simulink subsystem "XinSVSF3rd"  (R2020b)
settings: Solver=VariableStepAuto  StartTime=0.0  StopTime=10.0  RelTol=1e-3
values from neighbouring files (symbols this model uses):
  DeltaT = 0.1    [IMM_SVSF_VBL_init.m]
  Eta = 1    [IMM_SVSF_VBL_init.m]
  Gamma = .38    (= 0.38)    [IMM_SVSF_VBL_init.m]
  Psi = 3.2    [IMM_SVSF_VBL_init.m]
  Q = diag([1e-8,1e-8,1e-8,1e-10,1e-10,1e-10])    [IMM_SVSF_VBL_init.m]
  R = [.5e-2 0;0  9.5e-2]    [IMM_SVSF_VBL_init.m]
undefined symbols (not defined in the file or in its folder): A
libraries: dspmtrx3 x4, dspinverses x1
settings Model: Creator=Sara  LastModifiedBy=Sara

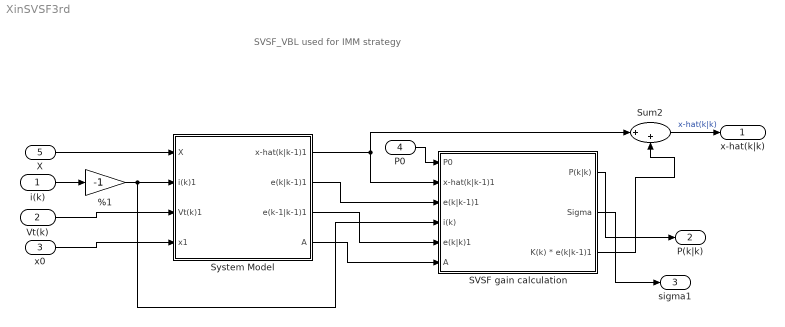
== system XinSVSF3rd ==
  note: SVSF_VBL used for IMM strategy
  i(k) : Inport
  Vt(k) : Inport  Port=2
  x0 : Inport  Port=3
  P0 : Inport  Port=4
  X : Inport  Port=5
  %1 : Gain  Gain=-1  SampleTime=DeltaT
  SVSF gain calculation : Subsystem
  Sum2 : Sum  Inputs=|++  SampleTime=DeltaT
  System Model : Subsystem
  x-hat(k|k) : Outport  VectorParamsAs1DForOutWhenUnconnected=off
  P(k|k) : Outport  Port=2
  sigma1 : Outport  Port=3
  wires:
  System Model/2(e(k|k-1)1) -> SVSF gain calculation/3(e(k|k-1)1)
  P0/1 -> SVSF gain calculation/1(P0)
  System Model/1(x-hat(k|k-1)1) -> SVSF gain calculation/2(x-hat(k|k-1)1), Sum2/1
  SVSF gain calculation/2(Sigma) -> sigma1/1
  System Model/3(e(k-1|k-1)1) -> SVSF gain calculation/5(e(k|k)1)
  SVSF gain calculation/3(K(k) * e(k|k-1)1) -> Sum2/2
  Sum2/1 -> x-hat(k|k)/1  "x-hat(k|k)"
  Vt(k)/1 -> System Model/3(Vt(k)1)
  SVSF gain calculation/1(P(k|k)) -> P(k|k)/1
  %1/1 -> System Model/2(i(k)1), SVSF gain calculation/4(i(k))
  x0/1 -> System Model/4(x1)
  System Model/4(A) -> SVSF gain calculation/6(A)
  X/1 -> System Model/1(X)
  i(k)/1 -> %1/1

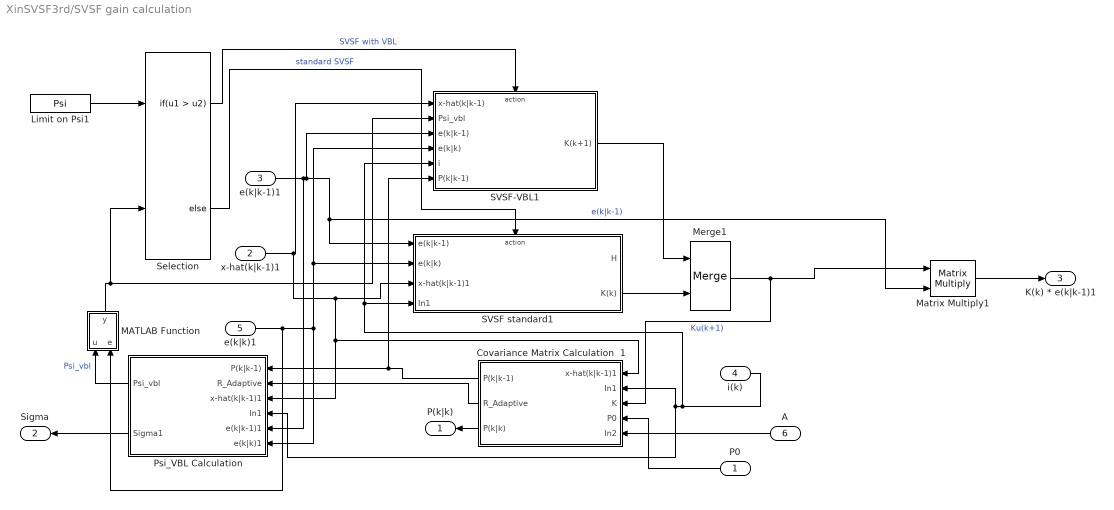
== system XinSVSF3rd/SVSF gain calculation ==
  P0 : Inport
  x-hat(k|k-1)1 : Inport  Port=2
  e(k|k-1)1 : Inport  Port=3
  i(k) : Inport  Port=4
  e(k|k)1 : Inport  Port=5
  A : Inport  Port=6
  " SVSF-VBL1" : Subsystem  TreatAsAtomicUnit=on
  " Selection" : If  NumInputs=2  IfExpression=u1 > u2
  Covariance Matrix Calculation  1 : Subsystem
  Limit on Psi1 : Constant  Value=Psi  SampleTime=DeltaT
  MATLAB Function : MATLAB Function  TreatAsAtomicUnit=on
  Matrix Multiply1 : Product  Multiplication=Matrix(*)
  Merge1 : Merge
  Psi_VBL Calculation : Subsystem
  SVSF standard1 : Subsystem
  P(k|k) : Outport
  Sigma : Outport  Port=2
  K(k) * e(k|k-1)1 : Outport  Port=3
  wires:
  Psi_VBL Calculation/2(Sigma1) -> Sigma/1
  Covariance Matrix Calculation  1/3("P(k|k) ") -> P(k|k)/1
  P0/1 -> Covariance Matrix Calculation  1/4(P0)
  e(k|k-1)1/1 -> SVSF standard1/1(e(k|k-1)), Matrix Multiply1/2, " SVSF-VBL1"/3(e(k|k-1)), Psi_VBL Calculation/5(e(k|k-1)1)  "e(k|k-1)"
  Psi_VBL Calculation/1(Psi_vbl) -> MATLAB Function/1(u)  "Psi_vbl"
  Covariance Matrix Calculation  1/1(P(k|k-1)) -> " SVSF-VBL1"/6(P(k|k-1)), Psi_VBL Calculation/1(P(k|k-1))
  SVSF standard1/2(K(k)) -> Merge1/2
  Limit on Psi1/1 -> " Selection"/1
  e(k|k)1/1 -> SVSF standard1/2(e(k|k)), " SVSF-VBL1"/4(e(k|k)), Psi_VBL Calculation/6(e(k|k)1), MATLAB Function/2(e)
  " Selection"/2 -> SVSF standard1/Action  "standard SVSF"
  Merge1/1 -> Matrix Multiply1/1, Covariance Matrix Calculation  1/3(K)  "Ku(k+1)"
  " SVSF-VBL1"/1(K(k+1)) -> Merge1/1
  x-hat(k|k-1)1/1 -> SVSF standard1/3(x-hat(k|k-1)1), Covariance Matrix Calculation  1/1(x-hat(k|k-1)1), Psi_VBL Calculation/3(x-hat(k|k-1)1), " SVSF-VBL1"/1(x-hat(k|k-1))
  i(k)/1 -> Covariance Matrix Calculation  1/2(In1), Psi_VBL Calculation/4(In1), SVSF standard1/4(In1), " SVSF-VBL1"/5(i)
  Matrix Multiply1/1 -> K(k) * e(k|k-1)1/1
  " Selection"/1 -> " SVSF-VBL1"/Action  "SVSF with VBL"
  Covariance Matrix Calculation  1/2(R_Adaptive) -> Psi_VBL Calculation/2(R_Adaptive)
  MATLAB Function/1(y) -> " Selection"/2, " SVSF-VBL1"/2(Psi_vbl)
  A/1 -> Covariance Matrix Calculation  1/5(In2)

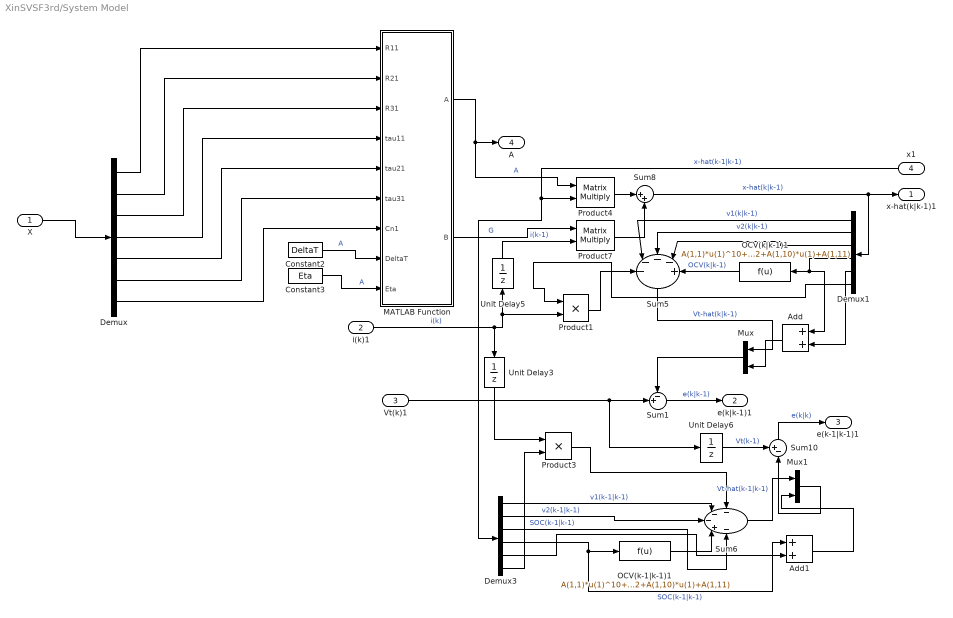
== system XinSVSF3rd/System Model ==
  X : Inport
  i(k)1 : Inport  Port=2
  Vt(k)1 : Inport  Port=3
  x1 : Inport  Port=4
  Add : Sum
  Add1 : Sum
  Constant2 : Constant  Value=DeltaT  SampleTime=DeltaT
  Constant3 : Constant  Value=Eta  SampleTime=DeltaT
  Demux : Demux  Outputs=7
  Demux1 : Demux  Outputs=6
  Demux3 : Demux  Outputs=6
  MATLAB Function : MATLAB Function  TreatAsAtomicUnit=on
  Mux : Mux  Inputs=2
  Mux1 : Mux  Inputs=2
  OCV(k-1|k-1)1 : Fcn  Expr=A(1,1)*u(1)^10+A(1,2)*u(1)^9+A(1,3)*u(1)^8+A(1,4)*u(1)^7+A(1,5)*u(1)^6+A(1,6)*u(1)^5+A(1,7)*u(1)^4+A(1,8)*u(1)^3+A(1,9)*u(1)^2+A(1,10)*u(1)+A(1,11)  SampleTime=DeltaT
  OCV(k|k-1)1 : Fcn  Expr=A(1,1)*u(1)^10+A(1,2)*u(1)^9+A(1,3)*u(1)^8+A(1,4)*u(1)^7+A(1,5)*u(1)^6+A(1,6)*u(1)^5+A(1,7)*u(1)^4+A(1,8)*u(1)^3+A(1,9)*u(1)^2+A(1,10)*u(1)+A(1,11)  SampleTime=DeltaT
  Product1 : Product
  Product3 : Product
  Product4 : Product  Multiplication=Matrix(*)  RndMeth=Zero  SampleTime=DeltaT
  Product7 : Product  Multiplication=Matrix(*)  RndMeth=Zero  SampleTime=DeltaT
  Sum1 : Sum  Inputs=-+|  SampleTime=DeltaT
  Sum10 : Sum  Inputs=+-|  SampleTime=DeltaT
  Sum5 : Sum  Inputs=----+  SampleTime=DeltaT
  Sum6 : Sum  Inputs=---+-  SampleTime=DeltaT
  Sum8 : Sum  Inputs=|++  SampleTime=DeltaT
  Unit Delay3 : UnitDelay  SampleTime=DeltaT  HasFrameUpgradeWarning=on
  Unit Delay5 : UnitDelay  SampleTime=DeltaT  HasFrameUpgradeWarning=on
  Unit Delay6 : UnitDelay  SampleTime=DeltaT  HasFrameUpgradeWarning=on
  x-hat(k|k-1)1 : Outport
  e(k|k-1)1 : Outport  Port=2
  e(k-1|k-1)1 : Outport  Port=3
  A : Outport  Port=4
  wires:
  Product1/1 -> Sum5/1
  Demux1/6 -> Product1/1
  Demux/7 -> MATLAB Function/7(Cn1)
  Demux/6 -> MATLAB Function/6(tau31)
  Demux/5 -> MATLAB Function/5(tau21)
  Demux/4 -> MATLAB Function/4(tau11)
  Demux/3 -> MATLAB Function/3(R31)
  Demux/2 -> MATLAB Function/2(R21)
  Demux/1 -> MATLAB Function/1(R11)
  X/1 -> Demux/1
  Sum6/1 -> Mux1/1  "Vt-hat(k-1|k-1)"
  x1/1 -> Product4/2, Demux3/1  "x-hat(k-1|k-1)"
  Demux1/5 -> Add/2
  Demux1/4 -> OCV(k|k-1)1/1, Add/1
  MATLAB Function/2(B) -> Product7/1  "G"
  Add1/1 -> Mux1/2
  Demux3/1 -> Sum6/2  "v1(k-1|k-1)"
  Sum1/1 -> e(k|k-1)1/1  "e(k|k-1)"
  Sum8/1 -> x-hat(k|k-1)1/1, Demux1/1  "x-hat(k|k-1)"
  Add/1 -> Mux/2
  Sum10/1 -> e(k-1|k-1)1/1  "e(k|k)"
  Sum5/1 -> Mux/1  "Vt-hat(k|k-1)"
  Mux1/1 -> Sum10/2
  Demux3/4 -> OCV(k-1|k-1)1/1, Add1/1  "SOC(k-1|k-1)"
  OCV(k|k-1)1/1 -> Sum5/5  "OCV(k|k-1)"
  Mux/1 -> Sum1/1
  Demux3/5 -> Add1/2
  Product3/1 -> Sum6/1
  Product4/1 -> Sum8/1
  Demux1/2 -> Sum5/3  "v2(k|k-1)"
  i(k)1/1 -> Unit Delay3/1, Unit Delay5/1, Product1/2  "i(k)"
  Unit Delay3/1 -> Product3/1
  MATLAB Function/1(A) -> A/1, Product4/1  "A"
  Unit Delay5/1 -> Product7/2  "i(k-1)"
  Product7/1 -> Sum8/2
  Vt(k)1/1 -> Sum1/2, Unit Delay6/1
  Unit Delay6/1 -> Sum10/1  "Vt(k-1)"
  Demux1/1 -> Sum5/2  "v1(k|k-1)"
  OCV(k-1|k-1)1/1 -> Sum6/4
  Demux3/6 -> Product3/2
  Demux3/2 -> Sum6/3  "v2(k-1|k-1)"
  Constant2/1 -> MATLAB Function/8(DeltaT)  "A"
  Constant3/1 -> MATLAB Function/9(Eta)  "A"
  Demux1/3 -> Sum5/4
  Demux3/3 -> Sum6/5  "SOC(k-1|k-1)"

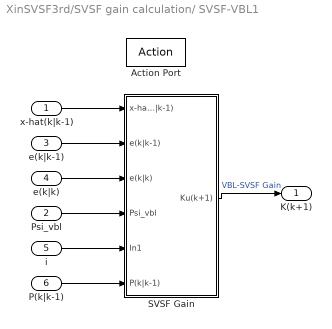
== system XinSVSF3rd/SVSF gain calculation/ SVSF-VBL1 ==
  x-hat(k|k-1) : Inport
  Psi_vbl : Inport  Port=2
  e(k|k-1) : Inport  Port=3
  e(k|k) : Inport  Port=4
  i : Inport  Port=5
  P(k|k-1) : Inport  Port=6
  Action Port : ActionPort
  SVSF Gain : Subsystem
  K(k+1) : Outport
  wires:
  P(k|k-1)/1 -> SVSF Gain/6(P(k|k-1))
  i/1 -> SVSF Gain/5(In1)
  e(k|k)/1 -> SVSF Gain/3(e(k|k))
  Psi_vbl/1 -> SVSF Gain/4(Psi_vbl)
  x-hat(k|k-1)/1 -> SVSF Gain/1(x-hat(k|k-1))
  e(k|k-1)/1 -> SVSF Gain/2(e(k|k-1))
  SVSF Gain/1(Ku(k+1)) -> K(k+1)/1  "VBL-SVSF Gain"

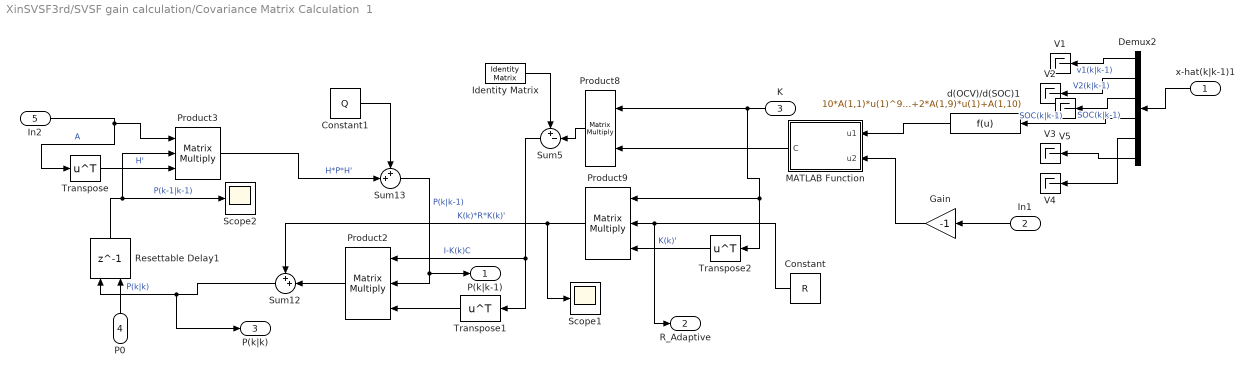
== system XinSVSF3rd/SVSF gain calculation/Covariance Matrix Calculation  1 ==
  x-hat(k|k-1)1 : Inport
  In1 : Inport  Port=2
  K : Inport  Port=3
  P0 : Inport  Port=4
  In2 : Inport  Port=5
  Constant : Constant  Value=R
  Constant1 : Constant  Value=Q
  Demux2 : Demux  Outputs=6
  Gain : Gain  Gain=-1
  Identity Matrix : dspmtrx3/Identity Matrix  Inherit=off  N=6  Ts=DeltaT  dataType=double  isSigned=on  wordLen=16  udDataType=sfix(16)  fracBitsMode=Best precision  numFracBits=15  OutDataTypeStr=double  LastOutDataTypeStr=double
  MATLAB Function : MATLAB Function  TreatAsAtomicUnit=on
  Product2 : Product  Inputs=3  Multiplication=Matrix(*)  RndMeth=Zero  SampleTime=DeltaT
  Product3 : Product  Inputs=3  Multiplication=Matrix(*)  RndMeth=Zero  SampleTime=DeltaT
  Product8 : Product  Multiplication=Matrix(*)  RndMeth=Zero  SampleTime=DeltaT
  Product9 : Product  Inputs=3  Multiplication=Matrix(*)  RndMeth=Zero  SampleTime=DeltaT
  Resettable Delay1 : Delay  DelayLength=1  InitialConditionSource=Input port  SampleTime=DeltaT
      settings: InputPortMap=u0,p4
  Scope1 : Scope
  Scope2 : Scope
  Sum12 : Sum  Inputs=++|  SampleTime=DeltaT
  Sum13 : Sum  Inputs=++|  SampleTime=DeltaT
  Sum5 : Sum  Inputs=+-|  SampleTime=DeltaT
  Transpose : Math  Operator=transpose  SignedPower=on  SaturateOnIntegerOverflow=on
  Transpose1 : Math  Operator=transpose  SignedPower=on  SaturateOnIntegerOverflow=on
  Transpose2 : Math  Operator=transpose  SignedPower=on  SaturateOnIntegerOverflow=on
  V{1..5} (5 alike) : Terminator
  d(OCV)/d(SOC)1 : Fcn  Expr=10*A(1,1)*u(1)^9+9*A(1,2)*u(1)^8+8*A(1,3)*u(1)^7+7*A(1,4)*u(1)^6+6*A(1,5)*u(1)^5+5*A(1,6)*u(1)^4+4*A(1,7)*u(1)^3+3*A(1,8)*u(1)^2+2*A(1,9)*u(1)+A(1,10)  SampleTime=DeltaT
  P(k|k-1) : Outport
  R_Adaptive : Outport  Port=2
  "P(k|k) " : Outport  Port=3
  wires:
  P0/1 -> Resettable Delay1/2
  Constant1/1 -> Sum13/1
  Constant/1 -> Product9/2, R_Adaptive/1
  K/1 -> Product9/1, Transpose2/1, Product8/1
  Sum13/1 -> Product2/2, P(k|k-1)/1  "P(k|k-1)"
  MATLAB Function/1(C) -> Product8/2
  Demux2/5 -> V4/1
  Demux2/6 -> V3/1
  Gain/1 -> MATLAB Function/2(u2)
  In1/1 -> Gain/1
  d(OCV)/d(SOC)1/1 -> MATLAB Function/1(u1)
  Demux2/2 -> V2/1  "V2(k|k-1)"
  Demux2/1 -> V1/1  "v1(k|k-1)"
  x-hat(k|k-1)1/1 -> Demux2/1
  Demux2/4 -> d(OCV)/d(SOC)1/1  "SOC(k|k-1)"
  In2/1 -> Product3/1, Transpose/1  "A"
  Transpose/1 -> Product3/3  "H'"
  Product2/1 -> Sum12/2
  Product3/1 -> Sum13/2  "H*P*H'"
  Sum5/1 -> Product2/1, Transpose1/1  "I-K(k)C"
  Sum12/1 -> Resettable Delay1/1, "P(k|k) "/1  "P(k|k)"
  Product8/1 -> Sum5/2
  Transpose2/1 -> Product9/3  "K(k)'"
  Product9/1 -> Sum12/1, Scope1/1  "K(k)*R*K(k)'"
  Resettable Delay1/1 -> Product3/2, Scope2/1  "P(k-1|k-1)"
  Transpose1/1 -> Product2/3
  Identity Matrix/1 -> Sum5/1
  Demux2/3 -> V5/1  "SOC(k|k-1)"

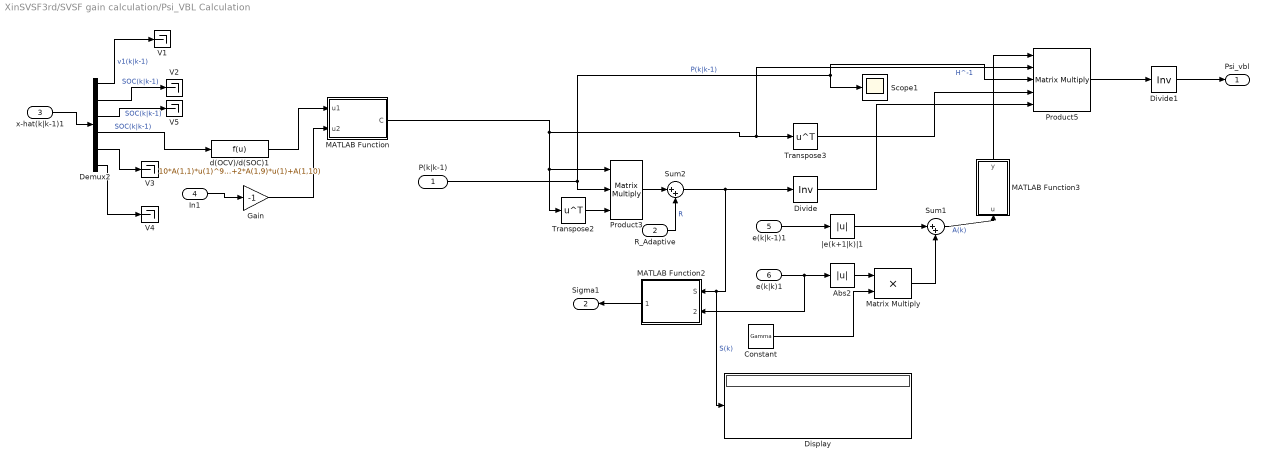
== system XinSVSF3rd/SVSF gain calculation/Psi_VBL Calculation ==
  P(k|k-1) : Inport
  R_Adaptive : Inport  Port=2
  x-hat(k|k-1)1 : Inport  Port=3
  In1 : Inport  Port=4
  e(k|k-1)1 : Inport  Port=5
  e(k|k)1 : Inport  Port=6
  Abs2 : Abs
  Constant : Constant  Value=Gamma
  Demux2 : Demux  Outputs=6
  Display : Display
  Divide : Product  Inputs=/  Multiplication=Matrix(*)  CollapseMode=Specified dimension
  Divide1 : Product  Inputs=/  Multiplication=Matrix(*)
  Gain : Gain  Gain=-1
  MATLAB Function : MATLAB Function  TreatAsAtomicUnit=on
  MATLAB Function2 : MATLAB Function  TreatAsAtomicUnit=on
  MATLAB Function3 : MATLAB Function  TreatAsAtomicUnit=on
  Matrix Multiply : Product
  Product3 : Product  Inputs=3  Multiplication=Matrix(*)  RndMeth=Zero
  Product5 : Product  Inputs=5  Multiplication=Matrix(*)  RndMeth=Zero
  Scope1 : Scope
  Sum1 : Sum  Inputs=|++
  Sum2 : Sum  Inputs=|++
  Transpose2 : Math  Operator=transpose  SaturateOnIntegerOverflow=on
  Transpose3 : Math  Operator=transpose  SaturateOnIntegerOverflow=on
  V{1..5} (5 alike) : Terminator
  d(OCV)/d(SOC)1 : Fcn  Expr=10*A(1,1)*u(1)^9+9*A(1,2)*u(1)^8+8*A(1,3)*u(1)^7+7*A(1,4)*u(1)^6+6*A(1,5)*u(1)^5+5*A(1,6)*u(1)^4+4*A(1,7)*u(1)^3+3*A(1,8)*u(1)^2+2*A(1,9)*u(1)+A(1,10)  SampleTime=DeltaT
  |e(k+1|k)|1 : Abs
  Psi_vbl : Outport
  Sigma1 : Outport  Port=2
  wires:
  P(k|k-1)/1 -> Scope1/1, Product5/3, Product3/2  "P(k|k-1)"
  Sum1/1 -> MATLAB Function3/1(u)  "A(k)"
  e(k|k)1/1 -> Abs2/1, MATLAB Function2/2(e_k_k_1)
  Sum2/1 -> Divide/1, MATLAB Function2/1(S), Display/1  "S(k)"
  Transpose2/1 -> Product3/3
  e(k|k-1)1/1 -> |e(k+1|k)|1/1
  MATLAB Function/1(C) -> Transpose3/1, Product5/2, Product3/1, Transpose2/1  "H^-1"
  Divide/1 -> Product5/5
  |e(k+1|k)|1/1 -> Sum1/1
  Transpose3/1 -> Product5/4
  Abs2/1 -> Matrix Multiply/1
  R_Adaptive/1 -> Sum2/2  "R"
  Matrix Multiply/1 -> Sum1/2
  MATLAB Function3/1(y) -> Product5/1
  Constant/1 -> Matrix Multiply/2
  Divide1/1 -> Psi_vbl/1
  Product5/1 -> Divide1/1
  Product3/1 -> Sum2/1
  MATLAB Function2/1(sigma2) -> Sigma1/1
  Demux2/6 -> V4/1
  Demux2/5 -> V3/1
  Gain/1 -> MATLAB Function/2(u2)
  In1/1 -> Gain/1
  Demux2/2 -> V2/1  "SOC(k|k-1)"
  d(OCV)/d(SOC)1/1 -> MATLAB Function/1(u1)
  Demux2/1 -> V1/1  "v1(k|k-1)"
  x-hat(k|k-1)1/1 -> Demux2/1
  Demux2/4 -> d(OCV)/d(SOC)1/1  "SOC(k|k-1)"
  Demux2/3 -> V5/1  "SOC(k|k-1)"

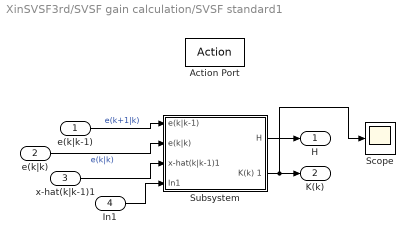
== system XinSVSF3rd/SVSF gain calculation/SVSF standard1 ==
  e(k|k-1) : Inport
  e(k|k) : Inport  Port=2
  x-hat(k|k-1)1 : Inport  Port=3
  In1 : Inport  Port=4
  Action Port : ActionPort
  Scope : Scope
  Subsystem : Subsystem
  H : Outport  VectorParamsAs1DForOutWhenUnconnected=off
  K(k) : Outport  Port=2
  wires:
  In1/1 -> Subsystem/4(In1)
  Subsystem/2(K(k) 1) -> K(k)/1, Scope/1
  Subsystem/1(H) -> H/1
  x-hat(k|k-1)1/1 -> Subsystem/3(x-hat(k|k-1)1)
  e(k|k)/1 -> Subsystem/2(e(k|k))  "e(k|k)"
  e(k|k-1)/1 -> Subsystem/1(e(k|k-1))  "e(k+1|k)"

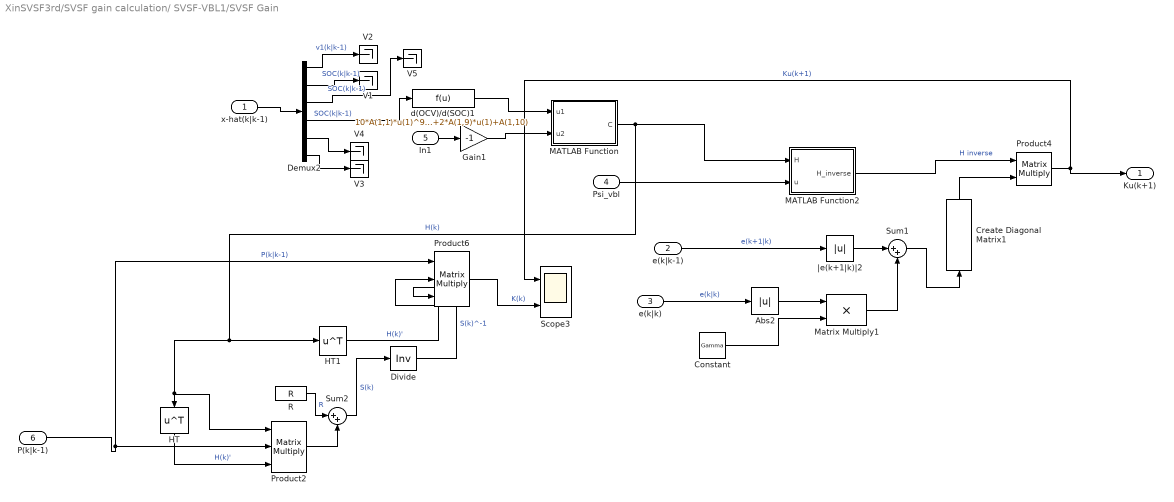
== system XinSVSF3rd/SVSF gain calculation/ SVSF-VBL1/SVSF Gain ==
  x-hat(k|k-1) : Inport
  e(k|k-1) : Inport  Port=2
  e(k|k) : Inport  Port=3
  Psi_vbl : Inport  Port=4
  In1 : Inport  Port=5
  P(k|k-1) : Inport  Port=6
  Abs2 : Abs
  Constant : Constant  Value=Gamma  SampleTime=DeltaT
  Create Diagonal Matrix1 : dspmtrx3/Create Diagonal Matrix
      settings: SourceProductBaseCode=DS
  Demux2 : Demux  Outputs=6
  Divide : Product  Inputs=/  Multiplication=Matrix(*)  SampleTime=DeltaT
  Gain1 : Gain  Gain=-1
  HT : Math  Operator=transpose  SignedPower=on  SaturateOnIntegerOverflow=on
  HT1 : Math  Operator=transpose  SignedPower=on  SaturateOnIntegerOverflow=on
  MATLAB Function : MATLAB Function  TreatAsAtomicUnit=on
  MATLAB Function2 : MATLAB Function  TreatAsAtomicUnit=on
  Matrix Multiply1 : Product
  Product2 : Product  Inputs=3  Multiplication=Matrix(*)  RndMeth=Zero  SampleTime=DeltaT
  Product4 : Product  Multiplication=Matrix(*)  RndMeth=Zero
  Product6 : Product  Inputs=3  Multiplication=Matrix(*)  RndMeth=Zero  SampleTime=DeltaT
  R : Constant  Value=R  SampleTime=DeltaT
  Scope3 : Scope  NumInputPorts=2
  Sum1 : Sum  Inputs=|++
  Sum2 : Sum  Inputs=|++  SampleTime=DeltaT
  V{1..5} (5 alike) : Terminator
  d(OCV)/d(SOC)1 : Fcn  Expr=10*A(1,1)*u(1)^9+9*A(1,2)*u(1)^8+8*A(1,3)*u(1)^7+7*A(1,4)*u(1)^6+6*A(1,5)*u(1)^5+5*A(1,6)*u(1)^4+4*A(1,7)*u(1)^3+3*A(1,8)*u(1)^2+2*A(1,9)*u(1)+A(1,10)  SampleTime=DeltaT
  |e(k+1|k)|2 : Abs
  Ku(k+1) : Outport
  wires:
  Product6/1 -> Scope3/2  "K(k)"
  Product4/1 -> Ku(k+1)/1, Scope3/1  "Ku(k+1)"
  R/1 -> Sum2/1  "R"
  MATLAB Function/1(C) -> MATLAB Function2/1(H), HT1/1, HT/1, Product2/1  "H(k)"
  Divide/1 -> Product6/3  "S(k)^-1"
  Sum2/1 -> Divide/1  "S(k)"
  P(k|k-1)/1 -> Product2/2, Product6/1  "P(k|k-1)"
  Product2/1 -> Sum2/2
  HT1/1 -> Product6/2  "H(k)'"
  HT/1 -> Product2/3  "H(k)'"
  e(k|k)/1 -> Abs2/1  "e(k|k)"
  Abs2/1 -> Matrix Multiply1/1
  e(k|k-1)/1 -> |e(k+1|k)|2/1  "e(k+1|k)"
  Matrix Multiply1/1 -> Sum1/2
  |e(k+1|k)|2/1 -> Sum1/1
  Constant/1 -> Matrix Multiply1/2
  Psi_vbl/1 -> MATLAB Function2/2(u)
  MATLAB Function2/1(H_inverse) -> Product4/1  "H inverse"
  Create Diagonal Matrix1/1 -> Product4/2
  Sum1/1 -> Create Diagonal Matrix1/1
  Demux2/5 -> V4/1
  Demux2/6 -> V3/1
  Gain1/1 -> MATLAB Function/2(u2)
  In1/1 -> Gain1/1
  Demux2/2 -> V1/1  "SOC(k|k-1)"
  d(OCV)/d(SOC)1/1 -> MATLAB Function/1(u1)
  Demux2/4 -> d(OCV)/d(SOC)1/1  "SOC(k|k-1)"
  Demux2/1 -> V2/1  "v1(k|k-1)"
  x-hat(k|k-1)/1 -> Demux2/1
  Demux2/3 -> V5/1  "SOC(k|k-1)"

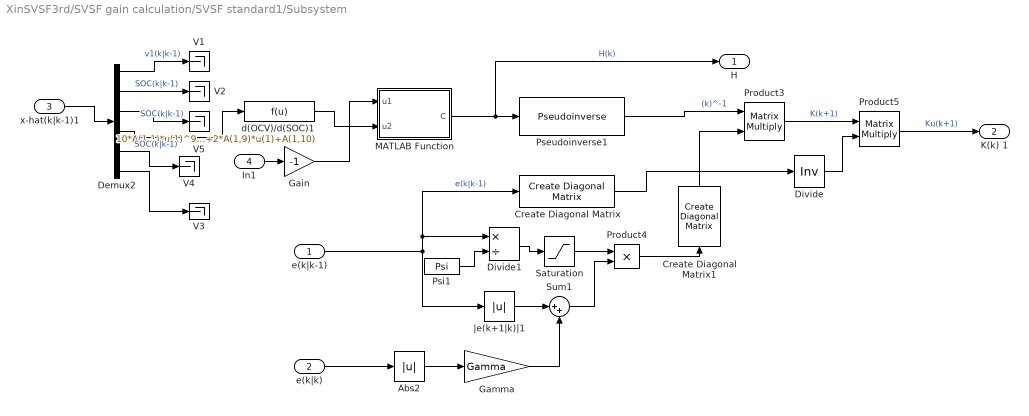
== system XinSVSF3rd/SVSF gain calculation/SVSF standard1/Subsystem ==
  e(k|k-1) : Inport
  e(k|k) : Inport  Port=2
  x-hat(k|k-1)1 : Inport  Port=3
  In1 : Inport  Port=4
  Abs2 : Abs  SampleTime=DeltaT
  Create Diagonal Matrix : dspmtrx3/Create Diagonal Matrix
      settings: SourceProductBaseCode=DS
  Create Diagonal Matrix1 : dspmtrx3/Create Diagonal Matrix
      settings: SourceProductBaseCode=DS
  Demux2 : Demux  Outputs=6
  Divide : Product  Inputs=/  Multiplication=Matrix(*)
  Divide1 : Product  Inputs=*/  SampleTime=DeltaT
  Gain : Gain  Gain=-1
  Gamma : Gain  Gain=Gamma  SampleTime=DeltaT
  MATLAB Function : MATLAB Function  TreatAsAtomicUnit=on
  Product3 : Product  Multiplication=Matrix(*)  RndMeth=Zero  SampleTime=DeltaT
  Product4 : Product  RndMeth=Zero  SampleTime=DeltaT
  Product5 : Product  Multiplication=Matrix(*)  RndMeth=Zero  SampleTime=DeltaT
  Pseudoinverse1 : dspinverses/Pseudoinverse  wanterr=off  SimulateUsing=Interpreted execution
      settings: SourceProductBaseCode=DS
  Psi1 : Constant  Value=Psi  SampleTime=DeltaT
  Saturation : Saturate  UpperLimit=1  LowerLimit=-1  SampleTime=DeltaT
  Sum1 : Sum  Inputs=|++  SampleTime=DeltaT
  V{1..5} (5 alike) : Terminator
  d(OCV)/d(SOC)1 : Fcn  Expr=10*A(1,1)*u(1)^9+9*A(1,2)*u(1)^8+8*A(1,3)*u(1)^7+7*A(1,4)*u(1)^6+6*A(1,5)*u(1)^5+5*A(1,6)*u(1)^4+4*A(1,7)*u(1)^3+3*A(1,8)*u(1)^2+2*A(1,9)*u(1)+A(1,10)  SampleTime=DeltaT
  |e(k+1|k)|1 : Abs  SampleTime=DeltaT
  H : Outport  VectorParamsAs1DForOutWhenUnconnected=off
  K(k) 1 : Outport  Port=2
  wires:
  Divide1/1 -> Saturation/1
  e(k|k-1)/1 -> |e(k+1|k)|1/1, Divide1/1, Create Diagonal Matrix/1  "e(k|k-1)"
  Psi1/1 -> Divide1/2
  Create Diagonal Matrix1/1 -> Product3/2
  Demux2/5 -> V4/1
  Demux2/6 -> V3/1
  Gain/1 -> MATLAB Function/1(u1)
  In1/1 -> Gain/1
  Demux2/2 -> V2/1  "SOC(k|k-1)"
  Create Diagonal Matrix/1 -> Divide/1
  x-hat(k|k-1)1/1 -> Demux2/1
  Demux2/1 -> V1/1  "v1(k|k-1)"
  Saturation/1 -> Product4/1
  Product3/1 -> Product5/1  "K(k+1)"
  Demux2/4 -> d(OCV)/d(SOC)1/1  "SOC(k|k-1)"
  Gamma/1 -> Sum1/2
  Product4/1 -> Create Diagonal Matrix1/1
  Pseudoinverse1/1 -> Product3/1  "(k)^-1"
  d(OCV)/d(SOC)1/1 -> MATLAB Function/2(u2)
  Sum1/1 -> Product4/2
  MATLAB Function/1(C) -> Pseudoinverse1/1, H/1  "H(k)"
  e(k|k)/1 -> Abs2/1
  Product5/1 -> K(k) 1/1  "Ku(k+1)"
  Divide/1 -> Product5/2
  Abs2/1 -> Gamma/1
  |e(k+1|k)|1/1 -> Sum1/1
  Demux2/3 -> V5/1  "SOC(k|k-1)"

== matlab function XinSVSF3rd/SVSF gain calculation/ SVSF-VBL1/SVSF Gain/MATLAB Function ==
  data: u1 input; u2 input; C output
function C = fcn(u1, u2)

C = [ -1 -1 -1 u1 0 u2;0 0 0 1 1 0];

== matlab function XinSVSF3rd/SVSF gain calculation/ SVSF-VBL1/SVSF Gain/MATLAB Function2 ==
  data: H_inverse output; H input; u input
function H_inverse = fcn(H, u)

%e = pinv(diag(u));
H_inverse = pinv(H)*(1/u);

== matlab function XinSVSF3rd/SVSF gain calculation/Covariance Matrix Calculation  1/MATLAB Function ==
  data: u1 input; u2 input; C output
function C = fcn(u1, u2)

C = [ -1 -1 -1 u1 0 u2;...
      0  0   0  1 1 0];

== matlab function XinSVSF3rd/SVSF gain calculation/MATLAB Function ==
  data: u input; y output; e input
function y  = fcn(u, e)

y = u(1,1);

if (abs(e(1)) > .0001) 
    cham = (e(1)- .0001)^2;
else 
    cham = 0; 
end

== matlab function XinSVSF3rd/SVSF gain calculation/Psi_VBL Calculation/MATLAB Function ==
  data: u1 input; u2 input; C output
function C = fcn(u1, u2)

C = [ -1 -1 -1 u1 0 u2;...
    0  0 0 1 1 0];

== matlab function XinSVSF3rd/SVSF gain calculation/Psi_VBL Calculation/MATLAB Function2 ==
  data: S input; e_k_k_1 input; sigma2 output
function sigma2  = fcn(S,e_k_k_1)

%sigma1 = (sqrt(abs(2*pi*S))^(-1))* exp(-e_k_k_1'*e_k_k_1*(2*inv(S)));
%  sigma2 =(exp(-0.5*e_k_k_1'*inv(S)*e_k_k_1))/(sqrt(abs(det(2*pi*S))));
%  sigma1 = normpdf(e_k_k_1,S);
 E = -1/2.*(e_k_k_1'*pinv(S)*e_k_k_1); 
 sigma2 = exp(E) / sqrt(abs(det(2*pi*S)));
end

== matlab function XinSVSF3rd/SVSF gain calculation/Psi_VBL Calculation/MATLAB Function3 ==
  data: u input; y output
function y = fcn(u)

y = pinv(diag(u));

== matlab function XinSVSF3rd/SVSF gain calculation/SVSF standard1/Subsystem/MATLAB Function ==
  data: u1 input; u2 input; C output
function C = fcn(u1, u2)

C = [ -1 -1 -1 u1 0 u2;0 0 0 1 1 0];

== matlab function XinSVSF3rd/System Model/MATLAB Function ==
  data: R11 input; R21 input; R31 input; tau11 input; tau21 input; tau31 input; Cn1 input; A output; DeltaT input; Eta input; B output
function [A,B] = fcn(R11, R21, R31, tau11, tau21, tau31, Cn1, DeltaT, Eta)
 C11 = tau11/R11;
 C21 = tau21/R21;
 C31 = tau31/R31;
C = Cn1 *3600;

A = [ 1-(DeltaT/(R11*C11)) 0 0 0 0 0;...
    0 1-(DeltaT/(R21*C21)) 0 0 0 0;...
    0 0 1-(DeltaT/(R31*C31)) 0 0 0;...
    0 0 0 1 0 0;...
    0 0 0 0 1 0;...
    0 0 0 0 0 1];
B = [ DeltaT/C11 ; DeltaT/C21; DeltaT/C31;-(Eta*DeltaT/C);0;0];
